simulink model "problem2"  (R2020b)
settings: Solver=VariableStepAuto  StartTime=0.0  StopTime=100  RelTol=1e-3
model workspace (MAT data in the model file):
  b = Simulink.Parameter
  b.Value = 200
  b.DataType = 'auto'
  b.Dimensions = [1 1]
  k1 = Simulink.Parameter
  k1.Value = 5000
  k1.DataType = 'auto'
  k1.Dimensions = [1 1]
  k2 = Simulink.Parameter
  k2.Value = 150
  k2.DataType = 'auto'
  k2.Dimensions = [1 1]
  m1 = Simulink.Parameter
  m1.Value = 400
  m1.DataType = 'auto'
  m1.Dimensions = [1 1]
  m2 = Simulink.Parameter
  m2.Value = 50
  m2.DataType = 'auto'
  m2.Dimensions = [1 1]
settings Model: Creator=Varun  LastModifiedBy=Varun

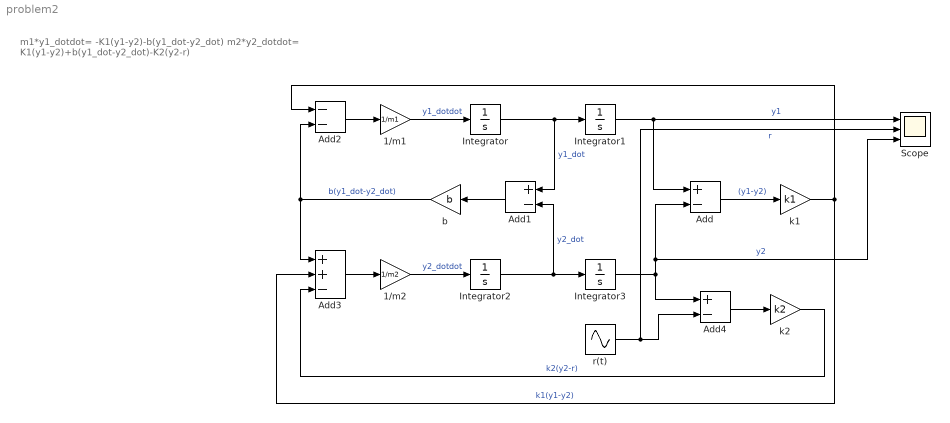
== system problem2 ==
  note: m1*y1_dotdot= -K1(y1-y2)-b(y1_dot-y2_dot)
      |
      | m2*y2_dotdot= K1(y1-y2)+b(y1_dot-y2_dot)-K2(y2-r)
  1/m1 : Gain  Gain=1/m1
  1/m2 : Gain  Gain=1/m2
  Add : Sum  Inputs=+-
  Add1 : Sum  Inputs=+-
  Add2 : Sum  Inputs=--
  Add3 : Sum  Inputs=++-
  Add4 : Sum  Inputs=+-
  Integrator{,1..3} (4 alike) : Integrator
  Scope : Scope  NumInputPorts=3
  b : Gain  Gain=b
  k1 : Gain  Gain=k1
  k2 : Gain  Gain=k2
  r(t) : Sin  Amplitude=0.05  Frequency=10  SampleTime=0
  wires:
  Integrator/1 -> Add1/1, Integrator1/1  "y1_dot"
  Integrator2/1 -> Add1/2, Integrator3/1  "y2_dot"
  Integrator1/1 -> Add/1, Scope/1  "y1"
  Integrator3/1 -> Scope/3, Add/2, Add4/1  "y2"
  Add/1 -> k1/1  "(y1-y2)"
  Add1/1 -> b/1
  Add2/1 -> 1/m1/1
  Add3/1 -> 1/m2/1
  b/1 -> Add3/1, Add2/2  "b(y1_dot-y2_dot)"
  k1/1 -> Add3/2, Add2/1  "k1(y1-y2)"
  1/m1/1 -> Integrator/1  "y1_dotdot"
  r(t)/1 -> Scope/2, Add4/2  "r"
  Add4/1 -> k2/1
  k2/1 -> Add3/3  "k2(y2-r)"
  1/m2/1 -> Integrator2/1  "y2_dotdot"
